simulink model "simu_test_2x1spokodziala3"  (Simulink 7.7)
settings: Solver=ode3  StartTime=0.0  StopTime=20.0  FixedStep=0.01  RelTol=1e-3
libraries: fuzblock x2, simulink x1
settings Model: Creator=Marcin  LastModifiedBy=Marcin

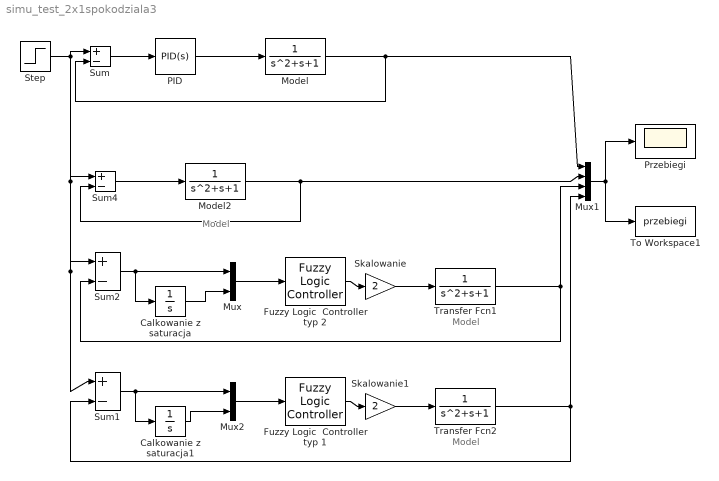
== system simu_test_2x1spokodziala3 ==
  note: Model
  note: Model
  note: Model
  Calkowanie z saturacja : Integrator  LimitOutput=on  UpperSaturationLimit=2  LowerSaturationLimit=-2
  Calkowanie z saturacja1 : Integrator  LimitOutput=on  UpperSaturationLimit=2  LowerSaturationLimit=-2
  Fuzzy Logic  Controller typ 1 : fuzblock/Fuzzy Logic  Controller  SystemSampleTime=-1  fis=fuzzy1
  Fuzzy Logic  Controller typ 2 : fuzblock/Fuzzy Logic  Controller  SystemSampleTime=-1  fis=fls
  Model : TransferFcn  Denominator=[1 1 1]
  Model2 : TransferFcn  Numerator=1  Denominator=[1 1 1]
  Mux : Mux  Inputs=2
  Mux1 : Mux
  Mux2 : Mux  Inputs=2
  PID : simulink/Continuous/PID Controller  SystemSampleTime=-1  Controller=PID  TimeDomain=Continuous-time  SampleTime=1  IntegratorMethod=Forward Euler  FilterMethod=Forward Euler  Form=Parallel  P=2  I=0.3  D=0.0001  N=100  InitialConditionSource=internal  InitialConditionForIntegrator=0  InitialConditionForFilter=0  ExternalReset=none  LimitOutput=off  UpperSaturationLimit=inf  LowerSaturationLimit=-inf  LinearizeAsGain=off  AntiWindupMode=none  Kb=1  TrackingMode=off  Kt=1  PParamMin=[]  PParamMax=[]  IParamMin=[]  IParamMax=[]  DParamMin=[]  DParamMax=[]  NParamMin=[]  NParamMax=[]  KbParamMin=[]  KbParamMax=[]  KtParamMin=[]  KtParamMax=[]  POutMin=[]  POutMax=[]  IOutMin=[]  IOutMax=[]  DOutMin=[]  DOutMax=[]  NOutMin=[]  NOutMax=[]  KbOutMin=[]  KbOutMax=[]  KtOutMin=[]  KtOutMax=[]  IntegratorOutMin=[]  IntegratorOutMax=[]  FilterOutMin=[]  FilterOutMax=[]  SumOutMin=[]  SumOutMax=[]  SumI1OutMin=[]  SumI1OutMax=[]  SumI2OutMin=[]  SumI2OutMax=[]  SumI3OutMin=[]  SumI3OutMax=[]  SumDOutMin=[]  SumDOutMax=[]  SaturationOutMin=[]  SaturationOutMax=[]  IntegratorContinuousStateAttributes=''  IntegratorStateMustResolveToSignalObject=off  IntegratorRTWStateStorageClass=Auto  FilterContinuousStateAttributes=''  FilterStateMustResolveToSignalObject=off  FilterRTWStateStorageClass=Auto
  Przebiegi : Scope
      settings: TimeRange=20  YMin=-0.5  YMax=2.75
  Skalowanie : Gain  Gain=2
  Skalowanie1 : Gain  Gain=2
  Step : Step  Time=0  SampleTime=0
  Sum{,1..2,4} (4 alike) : Sum  Inputs=|+-
  To Workspace1 : ToWorkspace  VariableName=przebiegi  SampleTime=-1  SaveFormat=Structure
  Transfer Fcn1 : TransferFcn  Denominator=[1 1 1]
  Transfer Fcn2 : TransferFcn  Denominator=[1 1 1]
  wires:
  Sum/1 -> PID/1
  Model/1 -> Sum/2, Mux1/1
  Step/1 -> Sum/1, Sum4/1, Sum2/1, Sum1/1
  PID/1 -> Model/1
  Transfer Fcn1/1 -> Sum2/2, Mux1/3
  Mux/1 -> Fuzzy Logic  Controller typ 2/1
  Model2/1 -> Sum4/2, Mux1/2
  Mux1/1 -> Przebiegi/1, To Workspace1/1
  Fuzzy Logic  Controller typ 2/1 -> Skalowanie/1
  Sum2/1 -> Mux/1, Calkowanie z saturacja/1
  Calkowanie z saturacja/1 -> Mux/2
  Sum4/1 -> Model2/1
  Skalowanie/1 -> Transfer Fcn1/1
  Transfer Fcn2/1 -> Sum1/2, Mux1/4
  Mux2/1 -> Fuzzy Logic  Controller typ 1/1
  Fuzzy Logic  Controller typ 1/1 -> Skalowanie1/1
  Sum1/1 -> Mux2/1, Calkowanie z saturacja1/1
  Calkowanie z saturacja1/1 -> Mux2/2
  Skalowanie1/1 -> Transfer Fcn2/1
